simulink model "bmw_roadster"  (R2018a)
settings: Solver=ode45  StartTime=0.0  StopTime=15  RelTol=1e-3  EnableMultiTasking=on
PreLoadFcn:
  | load gear_data;
  | FDR = 3.23;
  | AvgEngTorque = 222;
  | Loss = 0.8;
  | r_tire = 1.030;
  | m = 104.2;
  | Cd = 0.4;
  | rho = 2.377e-3;
  | h = 4.15;
  | w = 5.71;
settings Model: Creator=jrivitus  LastModifiedBy=bneiswan
settings DataIOCC: ExternalInput=[t, gear]  LimitDataPoints=on  LoadExternalInput=on  SaveFormat=Array
settings OptimizationCC: ExpressionDepthLimit=2147483647  LifeSpan=inf
settings DebuggingCC: UnderspecifiedInitializationDetection=Classic  MergeDetectMultiDrivingBlocksExec=none  ParameterPrecisionLossMsg=none  FcnCallInpInsideContextMsg=warning  AllowSymbolicDim=off  StateNameClashWarn=warning  SFUnexpectedBacktrackingDiag=warning  SFNoUnconditionalDefaultTransitionDiag=warning  SFExecutionAtInitializationDiag=none
settings HardwareCC: ProdBitPerPointer=32  ProdBitPerSizeT=32  ProdBitPerPtrDiffT=32  ProdLargestAtomicFloat=None  ProdIntDivRoundTo=Undefined  ProdEndianess=Unspecified  ProdWordSize=32  ProdHWDeviceType=32-bit Generic
settings ModelReferenceCC: PropagateSignalLabelsOutOfModel=off
settings CodeAppCC: StateflowObjectComments=on
settings GRTTargetCC: TargetLangStandard=C89/C90 (ANSI)  GeneratePreprocessorConditionals=Disable all  CombineOutputUpdateFcns=off  GRTInterface=on
settings ConfigComp: CovMetricSettings=dw  CovHtmlReporting=on  CovSaveCumulativeToWorkspaceVar=on  CovSaveSingleToWorkspaceVar=on  CovExternalEMLEnable=off  CovSFcnEnable=off

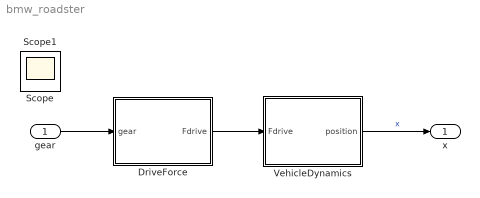
== system bmw_roadster ==
  gear : Inport
  DriveForce : Subsystem
  VehicleDynamics : Subsystem
      mask Display: image('carImg.jpg')
  x : Outport
  Scope : Scope
  Scope1 : Scope
  wires:
  DriveForce/1(Fdrive) -> VehicleDynamics/1(Fdrive)
  gear/1 -> DriveForce/1(gear)
  VehicleDynamics/1(position) -> x/1  "x"

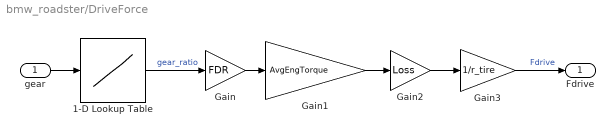
== system bmw_roadster/DriveForce ==
  gear : Inport
  1-D Lookup Table : Lookup_n-D  NumberOfTableDimensions=1  BreakpointsForDimension1=[1:5]  Table=[4.21 2.49 1.66 1.24 1.00]  InterpMethod=Flat  ExtrapMethod=Clip  RndMeth=Simplest  InputSameDT=on
  Gain : Gain  Gain=FDR
  Gain1 : Gain  Gain=AvgEngTorque
  Gain2 : Gain  Gain=Loss
  Gain3 : Gain  Gain=1/r_tire
  Fdrive : Outport
  wires:
  gear/1 -> 1-D Lookup Table/1
  1-D Lookup Table/1 -> Gain/1  "gear_ratio"
  Gain/1 -> Gain1/1
  Gain1/1 -> Gain2/1
  Gain2/1 -> Gain3/1
  Gain3/1 -> Fdrive/1  "Fdrive"

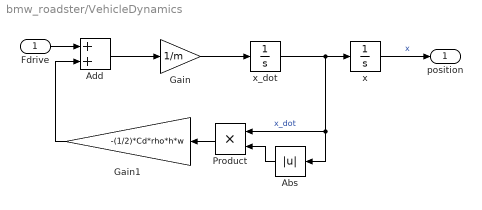
== system bmw_roadster/VehicleDynamics ==
  Fdrive : Inport
  Abs : Abs
  Add : Sum
  Gain : Gain  Gain=1/m
  Gain1 : Gain  Gain=-(1/2)*Cd*rho*h*w
  Product : Product  RndMeth=Zero
  x : Integrator
  x_dot : Integrator
  position : Outport
  wires:
  x_dot/1 -> x/1, Product/1, Abs/1  "x_dot"
  x/1 -> position/1  "x"
  Add/1 -> Gain/1
  Gain/1 -> x_dot/1
  Abs/1 -> Product/2
  Product/1 -> Gain1/1
  Gain1/1 -> Add/2
  Fdrive/1 -> Add/1
